simulink model "LVTresEspecies"  (R2020b)
settings: Solver=FixedStepAuto  StartTime=0.0  StopTime=20  FixedStep=0.01  RelTol=1e-3
values from neighbouring files (symbols this model uses):
  U1 = entradas(i)    [Curva_linealidad.m]    (also in FindEquations.m = ui(1); Horario.m = 10; Linealizar.m = ui(1) + delta; Untitled.m = 0)
  U2 = ui(2)    [Curva_linealidad.m]    (also in FindEquations.m; Horario.m = 0; Linealizar.m; Untitled.m = 20)
  U3 = ui(3)    [Curva_linealidad.m]    (also in FindEquations.m; Horario.m = 0; Linealizar.m; Untitled.m = 0)
settings Model: Creator=usuario  LastModifiedBy=sofia
settings DataIOCC: SaveOutput=off  SignalLogging=off  DSMLogging=off  SaveTime=off  ReturnWorkspaceOutputs=off

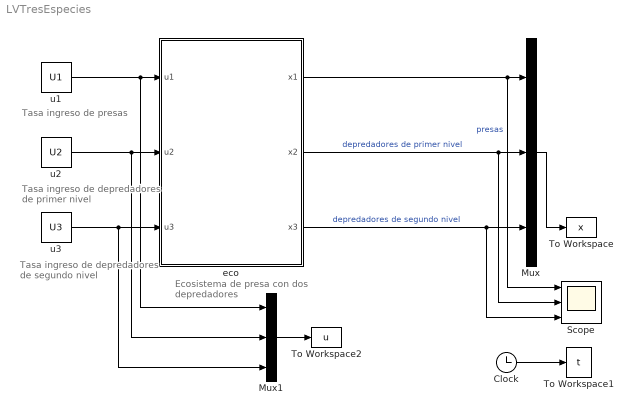
== system LVTresEspecies ==
  note: Ecosistema de presa con
      | dos depredadores
  note: Tasa ingreso de
      | presas
  note: Tasa ingreso de
      |  depredadores
      | de primer nivel
  note: Tasa ingreso de
      |  depredadores
      | de segundo nivel
  Clock : Clock
  Mux : Mux  Inputs=3
  Mux1 : Mux  Inputs=3
  Scope : Scope  NumInputPorts=3
  To Workspace : ToWorkspace  VariableName=x  SampleTime=-1
  To Workspace1 : ToWorkspace  VariableName=t  SampleTime=-1
  To Workspace2 : ToWorkspace  VariableName=u  SampleTime=-1
  eco : Subsystem  mask{ci=[794.9145      129.5644      12.95644], ri=[2.84         1.5        0.62], K=8640, ic=[0.22           0         0.1], pc=[0.02           0        0.03]}
      mask prompts: ci "Poblaciones iniciales [x10 x20 x30]"; ri "Tasas de crecimiento intrínseco  [r1 r2 r3]"; K "Capacidad de carga de las presas (K)"; ic "Constantes de interacción [a b c]"; pc "Constantes de proporcionalidad para la capacidad de carga [alpha beta chi]"
      mask init:
      | r1 = ri(1);
      | r2 = ri(2);
      | r3 = ri(3);
      | 
      | 
      | a = ic(1);
      | b = ic(2);
      | c = ic(3);
      | 
      | alpha = pc(1);
      | beta = pc(2);
      | chi = pc(3);
      | 
      | x10 = ci(1);
      | x20 = ci(2);
      | x30 = ci(3);
  u1 : Constant  Value=U1
  u2 : Constant  Value=U2
  u3 : Constant  Value=U3
  wires:
  u2/1 -> Mux1/2, eco/2(u2)
  eco/2("x2 ") -> Scope/2, Mux/2  "depredadores de primer nivel"
  u3/1 -> Mux1/3, eco/3(u3)
  u1/1 -> Mux1/1, eco/1(u1)
  Clock/1 -> To Workspace1/1
  eco/3("x3 ") -> Scope/3, Mux/3  "depredadores de segundo nivel"
  Mux/1 -> To Workspace/1
  eco/1("x1 ") -> Scope/1, Mux/1  "presas"
  Mux1/1 -> To Workspace2/1

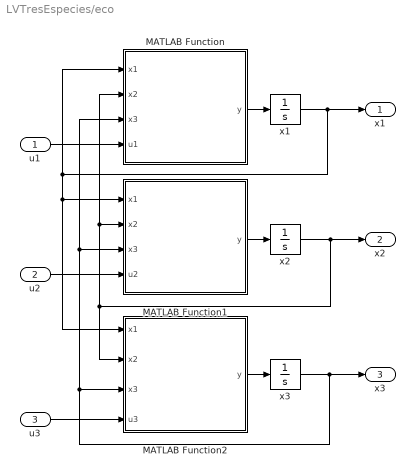
== system LVTresEspecies/eco ==
  u1 : Inport
  u2 : Inport  Port=2
  u3 : Inport  Port=3
  MATLAB Function : MATLAB Function  TreatAsAtomicUnit=on
  MATLAB Function1 : MATLAB Function  TreatAsAtomicUnit=on
  MATLAB Function2 : MATLAB Function  TreatAsAtomicUnit=on
  x1 : Integrator  InitialCondition=x10  LimitOutput=on  LowerSaturationLimit=0
  x2 : Integrator  InitialCondition=x20  LimitOutput=on  LowerSaturationLimit=0
  x3 : Integrator  InitialCondition=x30  LimitOutput=on  LowerSaturationLimit=0
  "x1 " : Outport
  "x2 " : Outport  Port=2
  "x3 " : Outport  Port=3
  wires:
  x1/1 -> "x1 "/1, MATLAB Function/1(x1), MATLAB Function2/1(x1), MATLAB Function1/1(x1)
  MATLAB Function1/1(y) -> x2/1
  u1/1 -> MATLAB Function/4(u1)
  x3/1 -> "x3 "/1, MATLAB Function1/3(x3), MATLAB Function/3(x3), MATLAB Function2/3(x3)
  MATLAB Function2/1(y) -> x3/1
  x2/1 -> "x2 "/1, MATLAB Function/2(x2), MATLAB Function1/2(x2), MATLAB Function2/2(x2)
  MATLAB Function/1(y) -> x1/1
  u2/1 -> MATLAB Function1/4(u2)
  u3/1 -> MATLAB Function2/4(u3)

== matlab function LVTresEspecies/eco/MATLAB Function ==
  data: r1 parameter; a parameter; b parameter; K parameter; y output; x1 input; x2 input; x3 input; u1 input
function y = fcn(r1,a,b,K,x1,x2,x3,u1)
y = r1*x1*(1-(x1/K))-a*x1*x2-b*x1*x3 + u1;

== matlab function LVTresEspecies/eco/MATLAB Function1 ==
  data: r2 parameter; alpha parameter; c parameter; y output; x1 input; x2 input; x3 input; u2 input
function y = fcn(r2,alpha,c,x1,x2,x3,u2)
    term=0;
    if alpha ~=0
        term = (x2/(alpha*x1));
        y = r2*x2*(1-term)-c*x2*x3+u2;
    else
        y = 0;
    end
end

== matlab function LVTresEspecies/eco/MATLAB Function2 ==
  data: r3 parameter; beta parameter; chi parameter; x1 input; x2 input; x3 input; y output; u3 input
function y = fcn(r3,beta,chi,x1,x2,x3,u3)
    term = 0;
    if not(beta == 0 && chi == 0)
        term = (x3/(beta*x1+chi*x2));
        y = r3*x3*(1-term)+u3;
    else
        y = 0;
    end
end
